simulink model "swc_1"  (R2023b)
settings: Solver=FixedStepDiscrete  StartTime=0.0  StopTime=10.0  FixedStep=0.01  RelTol=1e-3
settings Model: Creator=developer  LastModifiedBy=thabok
settings OptimizationCC: DefaultParameterBehavior=Inlined  EnhancedBackFolding=on  PassReuseOutputArgsAs=Individual arguments  ZeroExternalMemoryAtStartup=off  ZeroInternalMemoryAtStartup=off  OptimizeBlockOrder=speed  DifferentSizesBufferReuse=on  OptimizationCustomize=off  EfficientTunableParamExpr=on
settings DebuggingCC: ParameterTunabilityLossMsg=error
settings SFSimCC: MATLABDynamicMemAlloc=off
settings RTWCC: Description=Embedded Coder  SystemTargetFile=ert.tlc  GenCodeOnly=on  TemplateMakefile=ert_default_tmf
settings CodeAppCC: ForceParamTrailComments=on  IgnoreCustomStorageClasses=off  OperatorAnnotations=on  SimulinkDataObjDesc=on  SFDataObjDesc=on  InsertBlockDesc=on
settings ERTTargetCC: TargetLangStandard=C99 (ISO)  SupportAbsoluteTime=off  SupportNonFinite=off  SupportComplex=off  InlinedParameterPlacement=NonHierarchical  ERTCustomFileTemplate=example_file_process.tlc

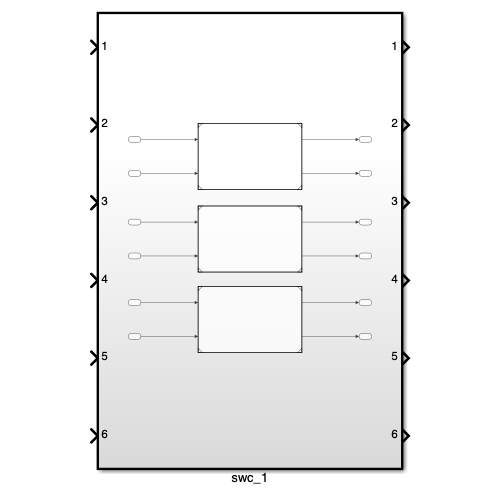
[thumbnail: Simulink's stored preview of the top-level diagram]
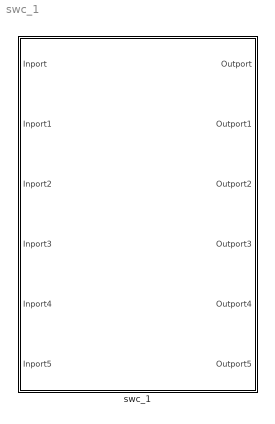
== system swc_1 ==
  swc_1 : Subsystem  TreatAsAtomicUnit=on
      settings: RTWSystemCode=Nonreusable function  RTWFcnNameOpts=Use subsystem name

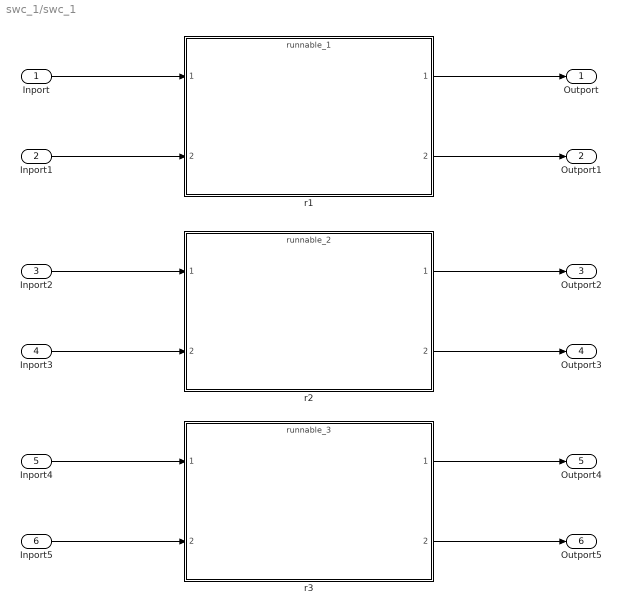
== system swc_1/swc_1 ==
  Inport : Inport
  Inport1 : Inport  Port=2
  Inport2 : Inport  Port=3
  Inport3 : Inport  Port=4
  Inport4 : Inport  Port=5
  Inport5 : Inport  Port=6
  r1 : ModelReference  ModelNameDialog=runnable_1.slx  SimulationMode=Normal  ModelReferenceVersion=3.0
  r2 : ModelReference  ModelNameDialog=runnable_2.slx  SimulationMode=Normal  ModelReferenceVersion=1.11
  r3 : ModelReference  ModelNameDialog=runnable_3.slx  SimulationMode=Normal  ModelReferenceVersion=3.0
  Outport : Outport
  Outport1 : Outport  Port=2
  Outport2 : Outport  Port=3
  Outport3 : Outport  Port=4
  Outport4 : Outport  Port=5
  Outport5 : Outport  Port=6
  wires:
  Inport/1 -> r1/1
  Inport1/1 -> r1/2
  Inport2/1 -> r2/1
  Inport3/1 -> r2/2
  Inport4/1 -> r3/1
  Inport5/1 -> r3/2
  r1/1 -> Outport/1
  r1/2 -> Outport1/1
  r2/1 -> Outport2/1
  r2/2 -> Outport3/1
  r3/1 -> Outport4/1
  r3/2 -> Outport5/1
